simulink subsystem "sistema_LTI"  (R2023b)
settings: Solver=VariableStepAuto  StartTime=0.0  StopTime=10.0  RelTol=1e-3
values from neighbouring files (symbols this model uses):
  b_eq = b_m + b_l/(r^2)    (= 2.19444444444e-05)    [constantes.m]    (also in test_polos_PID.m = b_m + b_l_nominal/(r^2))
  C_ts = 0.818    [constantes.m]
  k_l = g*(m*l_cm + m_l*l_l)    (= 2.4516625)    [constantes.m]
  lambda_m = 0.016    [constantes.m]
  Lq = 5.8e-3    (= 0.0058)    [constantes.m]
  P_p = 3    [constantes.m]
  r = 120    [constantes.m]
  R_sREF = 1.02    [constantes.m]
  R_ts_amb = 146.7    [constantes.m]
  T_s_inicial = 40    [constantes.m]
settings Model: Creator=nahue  LastModifiedBy=Nahuel

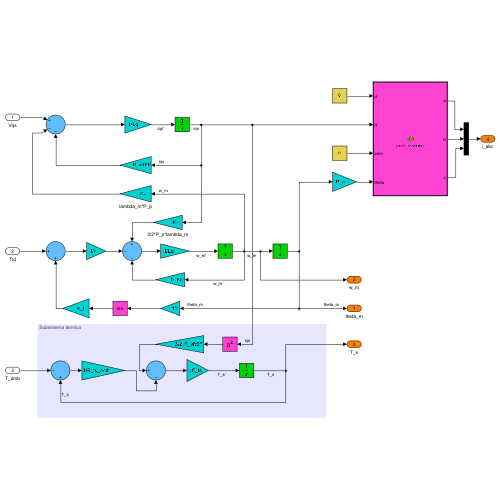
[thumbnail: Simulink's stored preview of the top-level diagram]
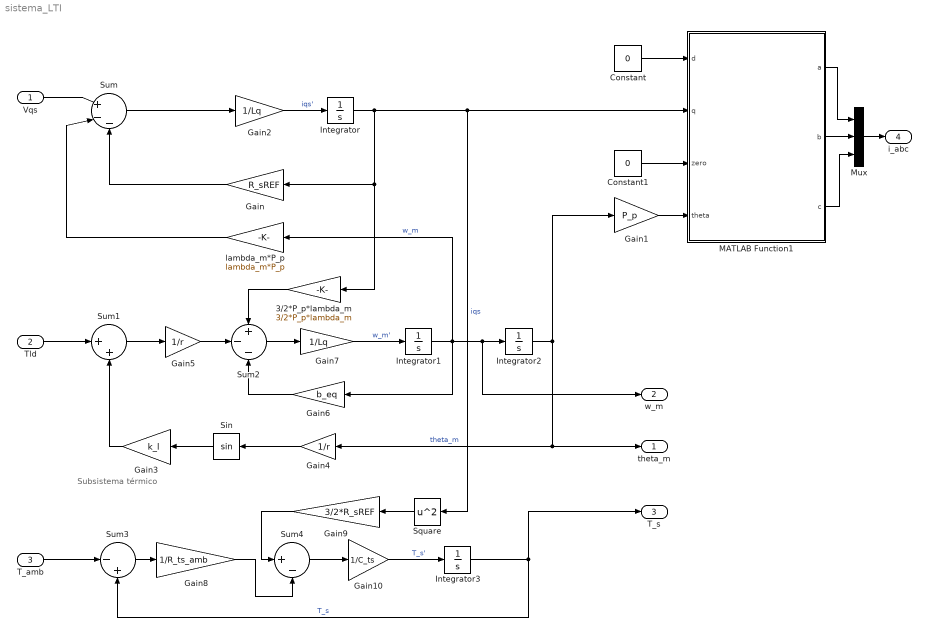
== system sistema_LTI ==
  note: Subsistema térmico
  Vqs : Inport
  Tld : Inport  Port=2
  T_amb : Inport  Port=3
  3/2*P_p*lambda_m : Gain  Gain=3/2*P_p*lambda_m
  Constant : Constant  Value=0
  Constant1 : Constant  Value=0
  Gain : Gain  Gain=R_sREF
  Gain1 : Gain  Gain=P_p
  Gain10 : Gain  Gain=1/C_ts
  Gain2 : Gain  Gain=1/Lq
  Gain3 : Gain  Gain=k_l
  Gain4 : Gain  Gain=1/r
  Gain5 : Gain  Gain=1/r
  Gain6 : Gain  Gain=b_eq
  Gain7 : Gain  Gain=1/Lq
  Gain8 : Gain  Gain=1/R_ts_amb
  Gain9 : Gain  Gain=3/2*R_sREF
  Integrator : Integrator
  Integrator1 : Integrator
  Integrator2 : Integrator
  Integrator3 : Integrator  InitialCondition=T_s_inicial
  MATLAB Function1 : MATLAB Function  TreatAsAtomicUnit=on
  Mux : Mux  Inputs=3
  Sin : Trigonometry
  Square : Math  Operator=square
  Sum : Sum  Inputs=|+--
  Sum1 : Sum  Inputs=|++
  Sum2 : Sum  Inputs=+--
  Sum3 : Sum  Inputs=|-+
  Sum4 : Sum  Inputs=|+-
  lambda_m*P_p : Gain  Gain=lambda_m*P_p
  theta_m : Outport
  w_m : Outport  Port=2
  T_s : Outport  Port=3
  i_abc : Outport  Port=4
  wires:
  Vqs/1 -> Sum/1
  Gain/1 -> Sum/3
  lambda_m*P_p/1 -> Sum/2
  Sum/1 -> Gain2/1
  Gain2/1 -> Integrator/1  "iqs'"
  Integrator/1 -> 3/2*P_p*lambda_m/1, Gain/1, Square/1, MATLAB Function1/2(q)  "iqs"
  Tld/1 -> Sum1/1
  Gain3/1 -> Sum1/2
  Sin/1 -> Gain3/1
  Gain4/1 -> Sin/1
  Sum1/1 -> Gain5/1
  Gain5/1 -> Sum2/2
  3/2*P_p*lambda_m/1 -> Sum2/1
  Gain6/1 -> Sum2/3
  Sum2/1 -> Gain7/1
  Gain7/1 -> Integrator1/1  "w_m'"
  Integrator1/1 -> w_m/1, Integrator2/1, Gain6/1, lambda_m*P_p/1  "w_m"
  Integrator2/1 -> Gain1/1, theta_m/1, Gain4/1  "theta_m"
  Gain1/1 -> MATLAB Function1/4(theta)
  Constant/1 -> MATLAB Function1/1(d)
  Constant1/1 -> MATLAB Function1/3(zero)
  T_amb/1 -> Sum3/1
  Sum3/1 -> Gain8/1
  Gain8/1 -> Sum4/2
  Gain9/1 -> Sum4/1
  Square/1 -> Gain9/1
  Sum4/1 -> Gain10/1
  Gain10/1 -> Integrator3/1  "T_s'"
  Integrator3/1 -> Sum3/2, T_s/1  "T_s"
  MATLAB Function1/1(a) -> Mux/1
  MATLAB Function1/2(b) -> Mux/2
  MATLAB Function1/3(c) -> Mux/3
  Mux/1 -> i_abc/1

== matlab function sistema_LTI/MATLAB Function1 ==
  data: d input; a output; q input; zero input; theta input; b output; c output
%% Transformación de Park Inversa
function [a, b, c] = park_inversa(d, q, zero, theta)
    % Transformación de Park Inversa usando una matriz
    % Entradas:
    %   d, q, z: Coordenadas en el marco rotatorio
    %   theta: Ángulo en radianes
    % Salidas:
    %   a, b, c: Valores trifásicos reconstruidos

    % Matriz de transformación inversa
    T = [
        cos(theta)             sin(theta)             1;
        cos(theta - 2*pi/3)    sin(theta - 2*pi/3)    1;
        cos(theta + 2*pi/3)    sin(theta + 2*pi/3)    1
    ];

    % Cálculo de los valores trifásicos
    abc = T * [d; q; zero];

    a = abc(1);
    b = abc(2);
    c = abc(3);
end
